simulink model "chap04"  (R2021a)
settings: Solver=FixedStepDiscrete  StartTime=0.0  StopTime=30  FixedStep=0.001  RelTol=1e-3
undefined symbols (not defined in the file): DiscIntNeverNeededParam
libraries: simulink x4
(part 6 of 7)

== system chap04/Subsystem/Subsystem7/Subsystem6 ==
  xx5 : Inport
  xx0 : Inport  Port=2
  xx3 : Inport  Port=3
  xx4 : Inport  Port=4
  vx5 : Inport  Port=5
  vx0 : Inport  Port=6
  vx3 : Inport  Port=7
  vx4 : Inport  Port=8
  Add : Sum
  Add1 : Sum  Inputs=-+
  Add10 : Sum  Inputs=-+
  Add2 : Sum  Inputs=+-
  Add4 : Sum  Inputs=-+
  Add5 : Sum  Inputs=+++
  Add6 : Sum  Inputs=+-
  Add8 : Sum  Inputs=+++
  Add9 : Sum  Inputs=+-
  Constant : Constant  Value=1.25
  Constant1 : Constant  Value=1.5
  Constant2 : Constant  Value=1.75
  Constant3 : Constant  Value=1.2
  Constant4 : Constant  Value=1.5
  Constant5 : Constant  Value=2.0
  Constant6 : Constant  Value=1.2
  Constant7 : Constant  Value=2.0
  Product{1,3..9} (8 alike) : Product
  utx : Outport
  wires:
  vx5/1 -> Add10/2, Add6/1, Add9/1
  vx4/1 -> Add10/1
  vx3/1 -> Add9/2
  xx3/1 -> Add2/2
  xx4/1 -> Add4/1
  Add/1 -> utx/1
  Add5/1 -> Product6/2
  Add2/1 -> Product5/1
  Product1/1 -> Add/2
  Constant2/1 -> Product1/1
  Constant/1 -> Product6/1
  Product6/1 -> Add/1
  Constant4/1 -> Product5/2
  xx5/1 -> Add1/2, Add4/2, Add2/1
  Add4/1 -> Product4/2
  Constant3/1 -> Product4/1
  Product5/1 -> Add5/3
  Product4/1 -> Add5/2
  Add8/1 -> Product1/2
  Constant6/1 -> Product8/1
  Add10/1 -> Product8/2
  Constant1/1 -> Product9/2
  Add9/1 -> Product9/1
  Product8/1 -> Add8/1
  Product9/1 -> Add8/2
  Constant7/1 -> Product3/1
  Add1/1 -> Product3/2
  xx0/1 -> Add1/1
  Product3/1 -> Add5/1
  Product7/1 -> Add8/3
  Add6/1 -> Product7/1
  Constant5/1 -> Product7/2
  vx0/1 -> Add6/2

== system chap04/Subsystem/Subsystem9/L+B ==
  Add : Sum
  Constant1 : Constant  Value=|
      | [2.7 0 0 0 0 0
      |      0 3.0 0 0 0 0
      |      0 0 3.0 0 0 0
      |      0 0 0 2.7 0 0
      |      0 0 0 0 2.7 0
      |      0 0 0 0 0 2.7]
  Constant2 : Constant  Value=|
      | [0.0 1.0 0.5 0.0 0.0 1.2
      |      1.0 0.0 0.0 0.5 0.0 1.5
      |      0.5 0.0 0.0 1.0 1.5 0.0
      |      0.0 0.5 1.0 0.0 1.2 0.0
      |      0.0 0.0 1.5 1.2 0.0 0.0
      |      1.2 1.5 0.0 0.0 0.0 0.0]
  Constant3 : Constant  Value=|
      | [0.0 0.0 0.0 0.0 0.0 0.0
      |      0.0 0.0 0.0 0.0 0.0 0.0
      |      0.0 0.0 0.0 0.0 0.0 0.0
      |      0.0 0.0 0.0 0.0 0.0 0.0
      |      0.0 0.0 0.0 0.0 2.0 0.0
      |      0.0 0.0 0.0 0.0 0.0 2.0]
  Subtract : Sum  Inputs=+-
  u : Outport
  wires:
  Constant2/1 -> Subtract/2
  Constant1/1 -> Subtract/1
  Subtract/1 -> Add/1
  Add/1 -> u/1
  Constant3/1 -> Add/2

== system chap04/Subsystem/Subsystem9/Subsystem1 ==
  xy3 : Inport
  xy1 : Inport  Port=2
  xy4 : Inport  Port=3
  xy5 : Inport  Port=4
  vy3 : Inport  Port=5
  vy1 : Inport  Port=6
  vy4 : Inport  Port=7
  vy5 : Inport  Port=8
  Add : Sum
  Add{1,4,6,8} (4 alike) : Sum  Inputs=-+
  Add2 : Sum  Inputs=+-
  Add5 : Sum  Inputs=+++
  Add7 : Sum  Inputs=+-
  Add9 : Sum  Inputs=+++
  Constant : Constant  Value=1.25
  Constant1 : Constant  Value=1.0
  Constant2 : Constant  Value=1.75
  Constant3 : Constant  Value=1.0
  Constant4 : Constant  Value=0.5
  Constant5 : Constant  Value=1.5
  Constant6 : Constant  Value=0.5
  Constant7 : Constant  Value=1.5
  Product{1,3..9} (8 alike) : Product
  p3y : Outport
  wires:
  Add9/1 -> Product1/2
  Product4/1 -> Add5/2
  Product5/1 -> Add5/3
  Constant3/1 -> Product4/1
  Add4/1 -> Product4/2
  xy3/1 -> Add1/2, Add4/2, Add2/1
  Constant4/1 -> Product5/2
  Product6/1 -> Add/1
  Constant/1 -> Product6/1
  Constant2/1 -> Product1/1
  Product1/1 -> Add/2
  Add2/1 -> Product5/1
  Add5/1 -> Product6/2
  Add/1 -> p3y/1
  xy4/1 -> Add4/1
  xy1/1 -> Add2/2
  xy5/1 -> Add1/1
  Constant5/1 -> Product3/1
  Add1/1 -> Product3/2
  Product3/1 -> Add5/1
  Product7/1 -> Add9/1
  Add6/1 -> Product7/2
  Constant7/1 -> Product7/1
  vy5/1 -> Add6/1
  vy1/1 -> Add7/2
  vy4/1 -> Add8/1
  Add7/1 -> Product9/1
  Constant6/1 -> Product9/2
  vy3/1 -> Add7/1, Add8/2, Add6/2
  Add8/1 -> Product8/2
  Constant1/1 -> Product8/1
  Product9/1 -> Add9/3
  Product8/1 -> Add9/2

== system chap04/Subsystem/Subsystem9/Subsystem2 ==
  xz3 : Inport
  xz1 : Inport  Port=2
  xz4 : Inport  Port=3
  xz5 : Inport  Port=4
  vz3 : Inport  Port=5
  vz1 : Inport  Port=6
  vz4 : Inport  Port=7
  vz5 : Inport  Port=8
  Add : Sum
  Add{1,4,6,8} (4 alike) : Sum  Inputs=-+
  Add2 : Sum  Inputs=+-
  Add5 : Sum  Inputs=+++
  Add7 : Sum  Inputs=+-
  Add9 : Sum  Inputs=+++
  Constant : Constant  Value=1.25
  Constant1 : Constant  Value=1.0
  Constant2 : Constant  Value=1.75
  Constant3 : Constant  Value=1.0
  Constant4 : Constant  Value=0.5
  Constant5 : Constant  Value=1.5
  Constant6 : Constant  Value=0.5
  Constant7 : Constant  Value=1.5
  Product{1,3..9} (8 alike) : Product
  p3z : Outport
  wires:
  Product8/1 -> Add9/2
  Product9/1 -> Add9/3
  Constant1/1 -> Product8/1
  Add8/1 -> Product8/2
  vz3/1 -> Add6/2, Add8/2, Add7/1
  Constant6/1 -> Product9/2
  Add7/1 -> Product9/1
  vz4/1 -> Add8/1
  vz1/1 -> Add7/2
  vz5/1 -> Add6/1
  Constant7/1 -> Product7/1
  Add6/1 -> Product7/2
  Product7/1 -> Add9/1
  Product3/1 -> Add5/1
  Add1/1 -> Product3/2
  Constant5/1 -> Product3/1
  xz5/1 -> Add1/1
  xz1/1 -> Add2/2
  xz4/1 -> Add4/1
  Add/1 -> p3z/1
  Add5/1 -> Product6/2
  Add2/1 -> Product5/1
  Product1/1 -> Add/2
  Constant2/1 -> Product1/1
  Constant/1 -> Product6/1
  Product6/1 -> Add/1
  Constant4/1 -> Product5/2
  xz3/1 -> Add2/1, Add4/2, Add1/2
  Add4/1 -> Product4/2
  Constant3/1 -> Product4/1
  Product5/1 -> Add5/3
  Product4/1 -> Add5/2
  Add9/1 -> Product1/2

== system chap04/Subsystem/Subsystem9/Subsystem3 ==
  xyk : Inport
  xy : Inport  Port=2
  vyk : Inport  Port=3
  vy : Inport  Port=4
  Add : Sum
  Add4 : Sum  Inputs=-+
  Add8 : Sum  Inputs=-+
  Constant : Constant  Value=1.25
  Constant1 : Constant  Value=1.75
  Product1 : Product
  Product6 : Product
  ey : Outport
  wires:
  vyk/1 -> Add8/2
  vy/1 -> Add8/1
  xy/1 -> Add4/1
  Add/1 -> ey/1
  Add4/1 -> Product6/2
  Product1/1 -> Add/2
  Constant1/1 -> Product1/1
  Constant/1 -> Product6/1
  Product6/1 -> Add/1
  xyk/1 -> Add4/2
  Add8/1 -> Product1/2

== system chap04/Subsystem/Subsystem9/Subsystem4 ==
  xzk : Inport
  xz : Inport  Port=2
  vzk : Inport  Port=3
  vz : Inport  Port=4
  Add : Sum
  Add4 : Sum  Inputs=-+
  Add8 : Sum  Inputs=-+
  Constant : Constant  Value=1.25
  Constant1 : Constant  Value=1.75
  Product1 : Product
  Product6 : Product
  ez : Outport
  wires:
  Add8/1 -> Product1/2
  xzk/1 -> Add4/2
  Product6/1 -> Add/1
  Constant/1 -> Product6/1
  Constant1/1 -> Product1/1
  Product1/1 -> Add/2
  Add4/1 -> Product6/2
  Add/1 -> ez/1
  xz/1 -> Add4/1
  vz/1 -> Add8/1
  vzk/1 -> Add8/2

== system chap04/Subsystem/Subsystem9/Subsystem5 ==
  xxk : Inport
  xx : Inport  Port=2
  vxk : Inport  Port=3
  vx : Inport  Port=4
  Add : Sum
  Add4 : Sum  Inputs=-+
  Add8 : Sum  Inputs=-+
  Constant : Constant  Value=1.25
  Constant1 : Constant  Value=1.75
  Product1 : Product
  Product6 : Product
  ex : Outport
  wires:
  Add8/1 -> Product1/2
  xxk/1 -> Add4/2
  Product6/1 -> Add/1
  Constant/1 -> Product6/1
  Constant1/1 -> Product1/1
  Product1/1 -> Add/2
  Add4/1 -> Product6/2
  Add/1 -> ex/1
  xx/1 -> Add4/1
  vx/1 -> Add8/1
  vxk/1 -> Add8/2

== system chap04/Subsystem/Subsystem9/Subsystem6 ==
  xx3 : Inport
  xx1 : Inport  Port=2
  xx4 : Inport  Port=3
  xx5 : Inport  Port=4
  vx3 : Inport  Port=5
  vx1 : Inport  Port=6
  vx4 : Inport  Port=7
  vx5 : Inport  Port=8
  Add : Sum
  Add{1,4,6,8} (4 alike) : Sum  Inputs=-+
  Add2 : Sum  Inputs=+-
  Add5 : Sum  Inputs=+++
  Add7 : Sum  Inputs=+-
  Add9 : Sum  Inputs=+++
  Constant : Constant  Value=1.25
  Constant1 : Constant  Value=1.0
  Constant2 : Constant  Value=1.75
  Constant3 : Constant  Value=1.0
  Constant4 : Constant  Value=0.5
  Constant5 : Constant  Value=1.5
  Constant6 : Constant  Value=0.5
  Constant7 : Constant  Value=1.5
  Product{1,3..9} (8 alike) : Product
  p3x : Outport
  wires:
  Product8/1 -> Add9/2
  Product9/1 -> Add9/3
  Constant1/1 -> Product8/1
  Add8/1 -> Product8/2
  vx3/1 -> Add6/2, Add8/2, Add7/1
  Constant6/1 -> Product9/2
  Add7/1 -> Product9/1
  vx4/1 -> Add8/1
  vx1/1 -> Add7/2
  vx5/1 -> Add6/1
  Constant7/1 -> Product7/1
  Add6/1 -> Product7/2
  Product7/1 -> Add9/1
  Product3/1 -> Add5/1
  Add1/1 -> Product3/2
  Constant5/1 -> Product3/1
  xx5/1 -> Add1/1
  xx1/1 -> Add2/2
  xx4/1 -> Add4/1
  Add/1 -> p3x/1
  Add5/1 -> Product6/2
  Add2/1 -> Product5/1
  Product1/1 -> Add/2
  Constant2/1 -> Product1/1
  Constant/1 -> Product6/1
  Product6/1 -> Add/1
  Constant4/1 -> Product5/2
  xx3/1 -> Add2/1, Add4/2, Add1/2
  Add4/1 -> Product4/2
  Constant3/1 -> Product4/1
  Product5/1 -> Add5/3
  Product4/1 -> Add5/2
  Add9/1 -> Product1/2

== system chap04/Subsystem1/Subsystem7/Subsystem1 ==
  Abs1 : Abs
  Add : Sum  Inputs=+++
  Constant : Constant  Value=0.8
  Constant1 : Constant  Value=0.1
  Constant3 : Constant  Value=0.1
  Delay1 : Delay
  Delay2 : Delay  DelayLength=1
  Product{1..4} (4 alike) : Product
  Random Number1 : RandomNumber  Mean=0.75  Variance=0.5  Seed=2  SampleTime=0.01
  Repeating Sequence Interpolated2 : simulink/Sources/Repeating Sequence Interpolated  OutValues=[0.5 0.25 0.4 0.35 0.1].'  TimeValues=[0 0.1 0.5 0.6 1].'  LookUpMeth=Use Input Nearest  tsamp=1  OutMin=[]  OutMax=[]  OutDataTypeStr=double  OutputDataTypeScalingMode=double  OutDataType=fixdt(0,8)  OutScaling=2^-10
  Scope : Scope
  Out2 : Outport
  wires:
  Delay1/1 -> Product2/1
  Delay2/1 -> Product1/1
  Constant/1 -> Product2/2
  Constant3/1 -> Product1/2
  Constant1/1 -> Product3/2
  Product3/1 -> Add/1
  Product1/1 -> Add/2
  Product2/1 -> Add/3
  Product4/1 -> Product3/1
  Add/1 -> Out2/1, Delay1/1, Delay2/1
  Abs1/1 -> Product4/1, Scope/1
  Random Number1/1 -> Abs1/1
  Repeating Sequence Interpolated2/1 -> Product4/2

== system chap04/Subsystem1/Subsystem7/Subsystem2 ==
  In2 : Inport
  Add : Sum  Inputs=+++
  Constant : Constant  Value=0.8
  Constant1 : Constant  Value=0.1
  Constant3 : Constant  Value=0.1
  Delay1 : Delay
  Delay2 : Delay  DelayLength=1
  Product1 : Product
  Product2 : Product
  Product3 : Product
  Out2 : Outport
  wires:
  Add/1 -> Delay2/1, Delay1/1, Out2/1
  In2/1 -> Product3/1
  Product2/1 -> Add/3
  Product1/1 -> Add/2
  Product3/1 -> Add/1
  Constant1/1 -> Product3/2
  Constant3/1 -> Product1/2
  Constant/1 -> Product2/2
  Delay2/1 -> Product1/1
  Delay1/1 -> Product2/1

== system chap04/Subsystem1/Subsystem7/Subsystem3 ==
  In2 : Inport
  Add : Sum  Inputs=+++
  Constant : Constant  Value=0.8
  Constant1 : Constant  Value=0.1
  Constant3 : Constant  Value=0.1
  Delay1 : Delay
  Delay2 : Delay  DelayLength=1
  Product1 : Product
  Product2 : Product
  Product3 : Product
  Out2 : Outport
  wires:
  Delay1/1 -> Product2/1
  Delay2/1 -> Product1/1
  Constant/1 -> Product2/2
  Constant3/1 -> Product1/2
  Constant1/1 -> Product3/2
  Product3/1 -> Add/1
  Product1/1 -> Add/2
  Product2/1 -> Add/3
  In2/1 -> Product3/1
  Add/1 -> Out2/1, Delay1/1, Delay2/1

== system chap04/Subsystem1/Subsystem7/Subsystem4 ==
  In2 : Inport
  Add : Sum  Inputs=+++
  Constant : Constant  Value=0.8
  Constant1 : Constant  Value=0.1
  Constant3 : Constant  Value=0.1
  Delay1 : Delay
  Delay2 : Delay  DelayLength=1
  Product1 : Product
  Product2 : Product
  Product3 : Product
  Out2 : Outport
  wires:
  Add/1 -> Delay2/1, Delay1/1, Out2/1
  In2/1 -> Product3/1
  Product2/1 -> Add/3
  Product1/1 -> Add/2
  Product3/1 -> Add/1
  Constant1/1 -> Product3/2
  Constant3/1 -> Product1/2
  Constant/1 -> Product2/2
  Delay2/1 -> Product1/1
  Delay1/1 -> Product2/1

== system chap04/Subsystem/Subsystem/Subsystem3/Subsystem ==
  e1 : Inport
  k3 : Inport  Port=2
  k4 : Inport  Port=3
  Add : Sum
  Constant3 : Constant  Value=-1
  Constant4 : Constant  Value=-1
  Discrete-Time Integrator1 : DiscreteIntegrator  SampleTime=-1  ICPrevOutput=DiscIntNeverNeededParam  ICPrevScaledInput=DiscIntNeverNeededParam
  Divide : Product  Inputs=*/
  MATLAB Function : MATLAB Function  TreatAsAtomicUnit=on
  Product3 : Product  Inputs=3
  Product5 : Product  Inputs=3
  z2 : Outport
  wires:
  Constant4/1 -> Product5/1
  Product5/1 -> Add/2
  Discrete-Time Integrator1/1 -> z2/1
  k3/1 -> Product3/3
  k4/1 -> Product5/3
  Divide/1 -> Add/1
  Add/1 -> Discrete-Time Integrator1/1
  Constant3/1 -> Product3/1
  e1/1 -> Product5/2, MATLAB Function/1(u), Product3/2
  MATLAB Function/1(y) -> Divide/2
  Product3/1 -> Divide/1

== system chap04/Subsystem/Subsystem/Subsystem3/Subsystem1 ==
  e1 : Inport
  k1 : Inport  Port=2
  Constant : Constant  Value=-1
  Divide : Product  Inputs=*/
  MATLAB Function : MATLAB Function  TreatAsAtomicUnit=on
  Product : Product  Inputs=3
  Out1 : Outport
  wires:
  e1/1 -> Product/2, MATLAB Function/1(u)
  Divide/1 -> Out1/1
  Constant/1 -> Product/1
  k1/1 -> Product/3
  MATLAB Function/1(y) -> Divide/2
  Product/1 -> Divide/1

== system chap04/Subsystem/Subsystem/Subsystem3/Subsystem2 ==
  e1 : Inport
  Constant1 : Constant  Value=0.2
  Discrete-Time Integrator1 : DiscreteIntegrator  gainval=1  InitialCondition=0.25  SampleTime=-1  ICPrevOutput=DiscIntNeverNeededParam  ICPrevScaledInput=DiscIntNeverNeededParam
  MATLAB Function : MATLAB Function  TreatAsAtomicUnit=on
  Product{,1..3,6} (5 alike) : Product
  Scope1 : Scope
  Sqrt : Sqrt  SaturateOnIntegerOverflow=on
  Square : Math  Operator=square  SaturateOnIntegerOverflow=on
  Subtract2 : Sum  Inputs=+-
  c1 : Constant  Value=0.3
  c2 : Constant  Value=0.3
  c3 : Constant  Value=0.5
  c4 : Constant  Value=0.5
  k1 : Outport
  k2 : Outport  Port=2
  k3 : Outport  Port=3
  k4 : Outport  Port=4
  wires:
  c2/1 -> Product/1
  Product/1 -> k2/1
  c3/1 -> Product1/1
  Product1/1 -> k3/1
  c4/1 -> Product2/1
  Product2/1 -> k4/1
  c1/1 -> Product3/1
  Product3/1 -> k1/1
  Sqrt/1 -> Product3/2
  Square/1 -> Product2/2
  e1/1 -> MATLAB Function/1(u)
  Product6/1 -> Subtract2/2
  MATLAB Function/1(y) -> Subtract2/1
  Subtract2/1 -> Discrete-Time Integrator1/1
  Constant1/1 -> Product6/1
  Discrete-Time Integrator1/1 -> Product6/2, Sqrt/1, Product/2, Square/1, Product1/2, Scope1/1

== system chap04/Subsystem/Subsystem/Subsystem3/Subsystem3 ==
  e1 : Inport
  k2 : Inport  Port=2
  Constant2 : Constant  Value=-1
  Product2 : Product  Inputs=3
  Out1 : Outport
  wires:
  Product2/1 -> Out1/1
  e1/1 -> Product2/2
  k2/1 -> Product2/3
  Constant2/1 -> Product2/1

== system chap04/Subsystem/Subsystem/Subsystem4/Subsystem ==
  zt3 : Inport
  Constant4 : Constant  Value=0
  Discrete-Time Integrator : DiscreteIntegrator  SampleTime=-1  UpperSaturationLimit=100  LowerSaturationLimit=-100  ICPrevOutput=DiscIntNeverNeededParam  ICPrevScaledInput=DiscIntNeverNeededParam
  Logical Operator : Logic  AllPortsSameDT=off  OutDataTypeStr=boolean
  MATLAB Function : MATLAB Function  TreatAsAtomicUnit=on
  Relational Operator : RelationalOperator  Operator===  OutDataTypeStr=boolean  RndMeth=Simplest
  Saturation : Saturate  UpperLimit=5  LowerLimit=-5
  Sign : Signum
  Sign1 : Signum
  Switch : Switch  Criteria=u2 > Threshold
  Out1 : Outport
  wires:
  MATLAB Function/1(y) -> Logical Operator/1
  Relational Operator/1 -> Logical Operator/2
  Constant4/1 -> Switch/1
  Sign1/1 -> Relational Operator/1
  zt3/1 -> Sign1/1, Switch/3
  Saturation/1 -> Out1/1, MATLAB Function/2(u2)
  Discrete-Time Integrator/1 -> Saturation/1, MATLAB Function/1(u1), Sign/1
  Sign/1 -> Relational Operator/2
  Logical Operator/1 -> Switch/2
  Switch/1 -> Discrete-Time Integrator/1

== system chap04/Subsystem/Subsystem/Subsystem7/Subsystem ==
  zt3 : Inport
  Constant4 : Constant  Value=0
  Discrete-Time Integrator : DiscreteIntegrator  SampleTime=-1  UpperSaturationLimit=100  LowerSaturationLimit=-100  ICPrevOutput=DiscIntNeverNeededParam  ICPrevScaledInput=DiscIntNeverNeededParam
  Logical Operator : Logic  AllPortsSameDT=off  OutDataTypeStr=boolean
  MATLAB Function : MATLAB Function  TreatAsAtomicUnit=on
  Relational Operator : RelationalOperator  Operator===  OutDataTypeStr=boolean  RndMeth=Simplest
  Saturation : Saturate  UpperLimit=5  LowerLimit=-5
  Sign : Signum
  Sign1 : Signum
  Switch : Switch  Criteria=u2 > Threshold
  Out1 : Outport
  wires:
  Switch/1 -> Discrete-Time Integrator/1
  Logical Operator/1 -> Switch/2
  Sign/1 -> Relational Operator/2
  Discrete-Time Integrator/1 -> Sign/1, MATLAB Function/1(u1), Saturation/1
  Saturation/1 -> MATLAB Function/2(u2), Out1/1
  zt3/1 -> Switch/3, Sign1/1
  Sign1/1 -> Relational Operator/1
  Constant4/1 -> Switch/1
  Relational Operator/1 -> Logical Operator/2
  MATLAB Function/1(y) -> Logical Operator/1

== system chap04/Subsystem/Subsystem/Subsystem8/Subsystem ==
  zt3 : Inport
  Constant4 : Constant  Value=0
  Discrete-Time Integrator : DiscreteIntegrator  SampleTime=-1  UpperSaturationLimit=100  LowerSaturationLimit=-100  ICPrevOutput=DiscIntNeverNeededParam  ICPrevScaledInput=DiscIntNeverNeededParam
  Logical Operator : Logic  AllPortsSameDT=off  OutDataTypeStr=boolean
  MATLAB Function : MATLAB Function  TreatAsAtomicUnit=on
  Relational Operator : RelationalOperator  Operator===  OutDataTypeStr=boolean  RndMeth=Simplest
  Saturation : Saturate  UpperLimit=5  LowerLimit=-5
  Sign : Signum
  Sign1 : Signum
  Switch : Switch  Criteria=u2 > Threshold
  Out1 : Outport
  wires:
  MATLAB Function/1(y) -> Logical Operator/1
  Relational Operator/1 -> Logical Operator/2
  Constant4/1 -> Switch/1
  Sign1/1 -> Relational Operator/1
  zt3/1 -> Sign1/1, Switch/3
  Saturation/1 -> Out1/1, MATLAB Function/2(u2)
  Discrete-Time Integrator/1 -> Saturation/1, MATLAB Function/1(u1), Sign/1
  Sign/1 -> Relational Operator/2
  Logical Operator/1 -> Switch/2
  Switch/1 -> Discrete-Time Integrator/1

== system chap04/Subsystem/Subsystem1/Subsystem3/Subsystem ==
  e1 : Inport
  k3 : Inport  Port=2
  k4 : Inport  Port=3
  Add : Sum
  Constant3 : Constant  Value=-1
  Constant4 : Constant  Value=-1
  Discrete-Time Integrator1 : DiscreteIntegrator  SampleTime=-1  ICPrevOutput=DiscIntNeverNeededParam  ICPrevScaledInput=DiscIntNeverNeededParam
  Divide : Product  Inputs=*/
  MATLAB Function : MATLAB Function  TreatAsAtomicUnit=on
  Product3 : Product  Inputs=3
  Product5 : Product  Inputs=3
  z2 : Outport
  wires:
  Constant4/1 -> Product5/1
  Product5/1 -> Add/2
  Discrete-Time Integrator1/1 -> z2/1
  k3/1 -> Product3/3
  k4/1 -> Product5/3
  Divide/1 -> Add/1
  Add/1 -> Discrete-Time Integrator1/1
  Constant3/1 -> Product3/1
  e1/1 -> Product5/2, MATLAB Function/1(u), Product3/2
  MATLAB Function/1(y) -> Divide/2
  Product3/1 -> Divide/1

== system chap04/Subsystem/Subsystem1/Subsystem3/Subsystem1 ==
  e1 : Inport
  k1 : Inport  Port=2
  Constant : Constant  Value=-1
  Divide : Product  Inputs=*/
  MATLAB Function : MATLAB Function  TreatAsAtomicUnit=on
  Product : Product  Inputs=3
  Out1 : Outport
  wires:
  e1/1 -> Product/2, MATLAB Function/1(u)
  Divide/1 -> Out1/1
  Constant/1 -> Product/1
  k1/1 -> Product/3
  MATLAB Function/1(y) -> Divide/2
  Product/1 -> Divide/1

== system chap04/Subsystem/Subsystem1/Subsystem3/Subsystem2 ==
  e1 : Inport
  Constant1 : Constant  Value=0.2
  Discrete-Time Integrator1 : DiscreteIntegrator  gainval=1  InitialCondition=0.25  SampleTime=-1  ICPrevOutput=DiscIntNeverNeededParam  ICPrevScaledInput=DiscIntNeverNeededParam
  MATLAB Function : MATLAB Function  TreatAsAtomicUnit=on
  Product{,1..3,6} (5 alike) : Product
  Scope1 : Scope
  Sqrt : Sqrt  SaturateOnIntegerOverflow=on
  Square : Math  Operator=square  SaturateOnIntegerOverflow=on
  Subtract2 : Sum  Inputs=+-
  c1 : Constant  Value=0.3
  c2 : Constant  Value=0.3
  c3 : Constant  Value=0.5
  c4 : Constant  Value=0.5
  k1 : Outport
  k2 : Outport  Port=2
  k3 : Outport  Port=3
  k4 : Outport  Port=4
  wires:
  c2/1 -> Product/1
  Product/1 -> k2/1
  c3/1 -> Product1/1
  Product1/1 -> k3/1
  c4/1 -> Product2/1
  Product2/1 -> k4/1
  c1/1 -> Product3/1
  Product3/1 -> k1/1
  Sqrt/1 -> Product3/2
  Square/1 -> Product2/2
  e1/1 -> MATLAB Function/1(u)
  Product6/1 -> Subtract2/2
  MATLAB Function/1(y) -> Subtract2/1
  Subtract2/1 -> Discrete-Time Integrator1/1
  Constant1/1 -> Product6/1
  Discrete-Time Integrator1/1 -> Product6/2, Sqrt/1, Product/2, Square/1, Product1/2, Scope1/1

== system chap04/Subsystem/Subsystem1/Subsystem3/Subsystem3 ==
  e1 : Inport
  k2 : Inport  Port=2
  Constant2 : Constant  Value=-1
  Product2 : Product  Inputs=3
  Out1 : Outport
  wires:
  Product2/1 -> Out1/1
  e1/1 -> Product2/2
  k2/1 -> Product2/3
  Constant2/1 -> Product2/1

== system chap04/Subsystem/Subsystem1/Subsystem4/Subsystem ==
  zt3 : Inport
  Constant4 : Constant  Value=0
  Discrete-Time Integrator : DiscreteIntegrator  SampleTime=-1  UpperSaturationLimit=100  LowerSaturationLimit=-100  ICPrevOutput=DiscIntNeverNeededParam  ICPrevScaledInput=DiscIntNeverNeededParam
  Logical Operator : Logic  AllPortsSameDT=off  OutDataTypeStr=boolean
  MATLAB Function : MATLAB Function  TreatAsAtomicUnit=on
  Relational Operator : RelationalOperator  Operator===  OutDataTypeStr=boolean  RndMeth=Simplest
  Saturation : Saturate  UpperLimit=5  LowerLimit=-5
  Sign : Signum
  Sign1 : Signum
  Switch : Switch  Criteria=u2 > Threshold
  Out1 : Outport
  wires:
  MATLAB Function/1(y) -> Logical Operator/1
  Relational Operator/1 -> Logical Operator/2
  Constant4/1 -> Switch/1
  Sign1/1 -> Relational Operator/1
  zt3/1 -> Sign1/1, Switch/3
  Saturation/1 -> Out1/1, MATLAB Function/2(u2)
  Discrete-Time Integrator/1 -> Saturation/1, MATLAB Function/1(u1), Sign/1
  Sign/1 -> Relational Operator/2
  Logical Operator/1 -> Switch/2
  Switch/1 -> Discrete-Time Integrator/1

== system chap04/Subsystem/Subsystem1/Subsystem7/Subsystem ==
  zt3 : Inport
  Constant4 : Constant  Value=0
  Discrete-Time Integrator : DiscreteIntegrator  SampleTime=-1  UpperSaturationLimit=100  LowerSaturationLimit=-100  ICPrevOutput=DiscIntNeverNeededParam  ICPrevScaledInput=DiscIntNeverNeededParam
  Logical Operator : Logic  AllPortsSameDT=off  OutDataTypeStr=boolean
  MATLAB Function : MATLAB Function  TreatAsAtomicUnit=on
  Relational Operator : RelationalOperator  Operator===  OutDataTypeStr=boolean  RndMeth=Simplest
  Saturation : Saturate  UpperLimit=5  LowerLimit=-5
  Sign : Signum
  Sign1 : Signum
  Switch : Switch  Criteria=u2 > Threshold
  Out1 : Outport
  wires:
  Switch/1 -> Discrete-Time Integrator/1
  Logical Operator/1 -> Switch/2
  Sign/1 -> Relational Operator/2
  Discrete-Time Integrator/1 -> Sign/1, MATLAB Function/1(u1), Saturation/1
  Saturation/1 -> MATLAB Function/2(u2), Out1/1
  zt3/1 -> Switch/3, Sign1/1
  Sign1/1 -> Relational Operator/1
  Constant4/1 -> Switch/1
  Relational Operator/1 -> Logical Operator/2
  MATLAB Function/1(y) -> Logical Operator/1

== system chap04/Subsystem/Subsystem1/Subsystem8/Subsystem ==
  zt3 : Inport
  Constant4 : Constant  Value=0
  Discrete-Time Integrator : DiscreteIntegrator  SampleTime=-1  UpperSaturationLimit=100  LowerSaturationLimit=-100  ICPrevOutput=DiscIntNeverNeededParam  ICPrevScaledInput=DiscIntNeverNeededParam
  Logical Operator : Logic  AllPortsSameDT=off  OutDataTypeStr=boolean
  MATLAB Function : MATLAB Function  TreatAsAtomicUnit=on
  Relational Operator : RelationalOperator  Operator===  OutDataTypeStr=boolean  RndMeth=Simplest
  Saturation : Saturate  UpperLimit=5  LowerLimit=-5
  Sign : Signum
  Sign1 : Signum
  Switch : Switch  Criteria=u2 > Threshold
  Out1 : Outport
  wires:
  MATLAB Function/1(y) -> Logical Operator/1
  Relational Operator/1 -> Logical Operator/2
  Constant4/1 -> Switch/1
  Sign1/1 -> Relational Operator/1
  zt3/1 -> Sign1/1, Switch/3
  Saturation/1 -> Out1/1, MATLAB Function/2(u2)
  Discrete-Time Integrator/1 -> Saturation/1, MATLAB Function/1(u1), Sign/1
  Sign/1 -> Relational Operator/2
  Logical Operator/1 -> Switch/2
  Switch/1 -> Discrete-Time Integrator/1

== system chap04/Subsystem/Subsystem2/Subsystem3/Subsystem ==
  e1 : Inport
  k3 : Inport  Port=2
  k4 : Inport  Port=3
  Add : Sum
  Constant3 : Constant  Value=-1
  Constant4 : Constant  Value=-1
  Discrete-Time Integrator1 : DiscreteIntegrator  SampleTime=-1  ICPrevOutput=DiscIntNeverNeededParam  ICPrevScaledInput=DiscIntNeverNeededParam
  Divide : Product  Inputs=*/
  MATLAB Function : MATLAB Function  TreatAsAtomicUnit=on
  Product3 : Product  Inputs=3
  Product5 : Product  Inputs=3
  z2 : Outport
  wires:
  Constant4/1 -> Product5/1
  Product5/1 -> Add/2
  Discrete-Time Integrator1/1 -> z2/1
  k3/1 -> Product3/3
  k4/1 -> Product5/3
  Divide/1 -> Add/1
  Add/1 -> Discrete-Time Integrator1/1
  Constant3/1 -> Product3/1
  e1/1 -> Product5/2, MATLAB Function/1(u), Product3/2
  MATLAB Function/1(y) -> Divide/2
  Product3/1 -> Divide/1

== system chap04/Subsystem/Subsystem2/Subsystem3/Subsystem1 ==
  e1 : Inport
  k1 : Inport  Port=2
  Constant : Constant  Value=-1
  Divide : Product  Inputs=*/
  MATLAB Function : MATLAB Function  TreatAsAtomicUnit=on
  Product : Product  Inputs=3
  Out1 : Outport
  wires:
  e1/1 -> Product/2, MATLAB Function/1(u)
  Divide/1 -> Out1/1
  Constant/1 -> Product/1
  k1/1 -> Product/3
  MATLAB Function/1(y) -> Divide/2
  Product/1 -> Divide/1

== system chap04/Subsystem/Subsystem2/Subsystem3/Subsystem2 ==
  e1 : Inport
  Constant1 : Constant  Value=0.2
  Discrete-Time Integrator1 : DiscreteIntegrator  gainval=1  InitialCondition=0.25  SampleTime=-1  ICPrevOutput=DiscIntNeverNeededParam  ICPrevScaledInput=DiscIntNeverNeededParam
  MATLAB Function : MATLAB Function  TreatAsAtomicUnit=on
  Product{,1..3,6} (5 alike) : Product
  Scope1 : Scope
  Sqrt : Sqrt  SaturateOnIntegerOverflow=on
  Square : Math  Operator=square  SaturateOnIntegerOverflow=on
  Subtract2 : Sum  Inputs=+-
  c1 : Constant  Value=0.3
  c2 : Constant  Value=0.3
  c3 : Constant  Value=0.5
  c4 : Constant  Value=0.5
  k1 : Outport
  k2 : Outport  Port=2
  k3 : Outport  Port=3
  k4 : Outport  Port=4
  wires:
  c2/1 -> Product/1
  Product/1 -> k2/1
  c3/1 -> Product1/1
  Product1/1 -> k3/1
  c4/1 -> Product2/1
  Product2/1 -> k4/1
  c1/1 -> Product3/1
  Product3/1 -> k1/1
  Sqrt/1 -> Product3/2
  Square/1 -> Product2/2
  e1/1 -> MATLAB Function/1(u)
  Product6/1 -> Subtract2/2
  MATLAB Function/1(y) -> Subtract2/1
  Subtract2/1 -> Discrete-Time Integrator1/1
  Constant1/1 -> Product6/1
  Discrete-Time Integrator1/1 -> Product6/2, Sqrt/1, Product/2, Square/1, Product1/2, Scope1/1

== system chap04/Subsystem/Subsystem2/Subsystem3/Subsystem3 ==
  e1 : Inport
  k2 : Inport  Port=2
  Constant2 : Constant  Value=-1
  Product2 : Product  Inputs=3
  Out1 : Outport
  wires:
  Product2/1 -> Out1/1
  e1/1 -> Product2/2
  k2/1 -> Product2/3
  Constant2/1 -> Product2/1

== system chap04/Subsystem/Subsystem2/Subsystem4/Subsystem ==
  zt3 : Inport
  Constant4 : Constant  Value=0
  Discrete-Time Integrator : DiscreteIntegrator  SampleTime=-1  UpperSaturationLimit=100  LowerSaturationLimit=-100  ICPrevOutput=DiscIntNeverNeededParam  ICPrevScaledInput=DiscIntNeverNeededParam
  Logical Operator : Logic  AllPortsSameDT=off  OutDataTypeStr=boolean
  MATLAB Function : MATLAB Function  TreatAsAtomicUnit=on
  Relational Operator : RelationalOperator  Operator===  OutDataTypeStr=boolean  RndMeth=Simplest
  Saturation : Saturate  UpperLimit=5  LowerLimit=-5
  Sign : Signum
  Sign1 : Signum
  Switch : Switch  Criteria=u2 > Threshold
  Out1 : Outport
  wires:
  MATLAB Function/1(y) -> Logical Operator/1
  Relational Operator/1 -> Logical Operator/2
  Constant4/1 -> Switch/1
  Sign1/1 -> Relational Operator/1
  zt3/1 -> Sign1/1, Switch/3
  Saturation/1 -> Out1/1, MATLAB Function/2(u2)
  Discrete-Time Integrator/1 -> Saturation/1, MATLAB Function/1(u1), Sign/1
  Sign/1 -> Relational Operator/2
  Logical Operator/1 -> Switch/2
  Switch/1 -> Discrete-Time Integrator/1

== system chap04/Subsystem/Subsystem2/Subsystem7/Subsystem ==
  zt3 : Inport
  Constant4 : Constant  Value=0
  Discrete-Time Integrator : DiscreteIntegrator  SampleTime=-1  UpperSaturationLimit=100  LowerSaturationLimit=-100  ICPrevOutput=DiscIntNeverNeededParam  ICPrevScaledInput=DiscIntNeverNeededParam
  Logical Operator : Logic  AllPortsSameDT=off  OutDataTypeStr=boolean
  MATLAB Function : MATLAB Function  TreatAsAtomicUnit=on
  Relational Operator : RelationalOperator  Operator===  OutDataTypeStr=boolean  RndMeth=Simplest
  Saturation : Saturate  UpperLimit=5  LowerLimit=-5
  Sign : Signum
  Sign1 : Signum
  Switch : Switch  Criteria=u2 > Threshold
  Out1 : Outport
  wires:
  Switch/1 -> Discrete-Time Integrator/1
  Logical Operator/1 -> Switch/2
  Sign/1 -> Relational Operator/2
  Discrete-Time Integrator/1 -> Sign/1, MATLAB Function/1(u1), Saturation/1
  Saturation/1 -> MATLAB Function/2(u2), Out1/1
  zt3/1 -> Switch/3, Sign1/1
  Sign1/1 -> Relational Operator/1
  Constant4/1 -> Switch/1
  Relational Operator/1 -> Logical Operator/2
  MATLAB Function/1(y) -> Logical Operator/1

== system chap04/Subsystem/Subsystem2/Subsystem8/Subsystem ==
  zt3 : Inport
  Constant4 : Constant  Value=0
  Discrete-Time Integrator : DiscreteIntegrator  SampleTime=-1  UpperSaturationLimit=100  LowerSaturationLimit=-100  ICPrevOutput=DiscIntNeverNeededParam  ICPrevScaledInput=DiscIntNeverNeededParam
  Logical Operator : Logic  AllPortsSameDT=off  OutDataTypeStr=boolean
  MATLAB Function : MATLAB Function  TreatAsAtomicUnit=on
  Relational Operator : RelationalOperator  Operator===  OutDataTypeStr=boolean  RndMeth=Simplest
  Saturation : Saturate  UpperLimit=5  LowerLimit=-5
  Sign : Signum
  Sign1 : Signum
  Switch : Switch  Criteria=u2 > Threshold
  Out1 : Outport
  wires:
  MATLAB Function/1(y) -> Logical Operator/1
  Relational Operator/1 -> Logical Operator/2
  Constant4/1 -> Switch/1
  Sign1/1 -> Relational Operator/1
  zt3/1 -> Sign1/1, Switch/3
  Saturation/1 -> Out1/1, MATLAB Function/2(u2)
  Discrete-Time Integrator/1 -> Saturation/1, MATLAB Function/1(u1), Sign/1
  Sign/1 -> Relational Operator/2
  Logical Operator/1 -> Switch/2
  Switch/1 -> Discrete-Time Integrator/1

== system chap04/Subsystem/Subsystem3/Subsystem3/Subsystem ==
  e1 : Inport
  k3 : Inport  Port=2
  k4 : Inport  Port=3
  Add : Sum
  Constant3 : Constant  Value=-1
  Constant4 : Constant  Value=-1
  Discrete-Time Integrator1 : DiscreteIntegrator  SampleTime=-1  ICPrevOutput=DiscIntNeverNeededParam  ICPrevScaledInput=DiscIntNeverNeededParam
  Divide : Product  Inputs=*/
  MATLAB Function : MATLAB Function  TreatAsAtomicUnit=on
  Product3 : Product  Inputs=3
  Product5 : Product  Inputs=3
  z2 : Outport
  wires:
  Constant4/1 -> Product5/1
  Product5/1 -> Add/2
  Discrete-Time Integrator1/1 -> z2/1
  k3/1 -> Product3/3
  k4/1 -> Product5/3
  Divide/1 -> Add/1
  Add/1 -> Discrete-Time Integrator1/1
  Constant3/1 -> Product3/1
  e1/1 -> Product5/2, MATLAB Function/1(u), Product3/2
  MATLAB Function/1(y) -> Divide/2
  Product3/1 -> Divide/1

== system chap04/Subsystem/Subsystem3/Subsystem3/Subsystem1 ==
  e1 : Inport
  k1 : Inport  Port=2
  Constant : Constant  Value=-1
  Divide : Product  Inputs=*/
  MATLAB Function : MATLAB Function  TreatAsAtomicUnit=on
  Product : Product  Inputs=3
  Out1 : Outport
  wires:
  e1/1 -> Product/2, MATLAB Function/1(u)
  Divide/1 -> Out1/1
  Constant/1 -> Product/1
  k1/1 -> Product/3
  MATLAB Function/1(y) -> Divide/2
  Product/1 -> Divide/1

== system chap04/Subsystem/Subsystem3/Subsystem3/Subsystem2 ==
  e1 : Inport
  Constant1 : Constant  Value=0.2
  Discrete-Time Integrator1 : DiscreteIntegrator  gainval=1  InitialCondition=0.25  SampleTime=-1  ICPrevOutput=DiscIntNeverNeededParam  ICPrevScaledInput=DiscIntNeverNeededParam
  MATLAB Function : MATLAB Function  TreatAsAtomicUnit=on
  Product{,1..3,6} (5 alike) : Product
  Scope1 : Scope
  Sqrt : Sqrt  SaturateOnIntegerOverflow=on
  Square : Math  Operator=square  SaturateOnIntegerOverflow=on
  Subtract2 : Sum  Inputs=+-
  c1 : Constant  Value=0.3
  c2 : Constant  Value=0.3
  c3 : Constant  Value=0.5
  c4 : Constant  Value=0.5
  k1 : Outport
  k2 : Outport  Port=2
  k3 : Outport  Port=3
  k4 : Outport  Port=4
  wires:
  c2/1 -> Product/1
  Product/1 -> k2/1
  c3/1 -> Product1/1
  Product1/1 -> k3/1
  c4/1 -> Product2/1
  Product2/1 -> k4/1
  c1/1 -> Product3/1
  Product3/1 -> k1/1
  Sqrt/1 -> Product3/2
  Square/1 -> Product2/2
  e1/1 -> MATLAB Function/1(u)
  Product6/1 -> Subtract2/2
  MATLAB Function/1(y) -> Subtract2/1
  Subtract2/1 -> Discrete-Time Integrator1/1
  Constant1/1 -> Product6/1
  Discrete-Time Integrator1/1 -> Product6/2, Sqrt/1, Product/2, Square/1, Product1/2, Scope1/1

== system chap04/Subsystem/Subsystem3/Subsystem3/Subsystem3 ==
  e1 : Inport
  k2 : Inport  Port=2
  Constant2 : Constant  Value=-1
  Product2 : Product  Inputs=3
  Out1 : Outport
  wires:
  Product2/1 -> Out1/1
  e1/1 -> Product2/2
  k2/1 -> Product2/3
  Constant2/1 -> Product2/1

== system chap04/Subsystem/Subsystem3/Subsystem4/Subsystem ==
  zt3 : Inport
  Constant4 : Constant  Value=0
  Discrete-Time Integrator : DiscreteIntegrator  SampleTime=-1  UpperSaturationLimit=100  LowerSaturationLimit=-100  ICPrevOutput=DiscIntNeverNeededParam  ICPrevScaledInput=DiscIntNeverNeededParam
  Logical Operator : Logic  AllPortsSameDT=off  OutDataTypeStr=boolean
  MATLAB Function : MATLAB Function  TreatAsAtomicUnit=on
  Relational Operator : RelationalOperator  Operator===  OutDataTypeStr=boolean  RndMeth=Simplest
  Saturation : Saturate  UpperLimit=5  LowerLimit=-5
  Sign : Signum
  Sign1 : Signum
  Switch : Switch  Criteria=u2 > Threshold
  Out1 : Outport
  wires:
  MATLAB Function/1(y) -> Logical Operator/1
  Relational Operator/1 -> Logical Operator/2
  Constant4/1 -> Switch/1
  Sign1/1 -> Relational Operator/1
  zt3/1 -> Sign1/1, Switch/3
  Saturation/1 -> Out1/1, MATLAB Function/2(u2)
  Discrete-Time Integrator/1 -> Saturation/1, MATLAB Function/1(u1), Sign/1
  Sign/1 -> Relational Operator/2
  Logical Operator/1 -> Switch/2
  Switch/1 -> Discrete-Time Integrator/1

== system chap04/Subsystem/Subsystem3/Subsystem7/Subsystem ==
  zt3 : Inport
  Constant4 : Constant  Value=0
  Discrete-Time Integrator : DiscreteIntegrator  SampleTime=-1  UpperSaturationLimit=100  LowerSaturationLimit=-100  ICPrevOutput=DiscIntNeverNeededParam  ICPrevScaledInput=DiscIntNeverNeededParam
  Logical Operator : Logic  AllPortsSameDT=off  OutDataTypeStr=boolean
  MATLAB Function : MATLAB Function  TreatAsAtomicUnit=on
  Relational Operator : RelationalOperator  Operator===  OutDataTypeStr=boolean  RndMeth=Simplest
  Saturation : Saturate  UpperLimit=5  LowerLimit=-5
  Sign : Signum
  Sign1 : Signum
  Switch : Switch  Criteria=u2 > Threshold
  Out1 : Outport
  wires:
  Switch/1 -> Discrete-Time Integrator/1
  Logical Operator/1 -> Switch/2
  Sign/1 -> Relational Operator/2
  Discrete-Time Integrator/1 -> Sign/1, MATLAB Function/1(u1), Saturation/1
  Saturation/1 -> MATLAB Function/2(u2), Out1/1
  zt3/1 -> Switch/3, Sign1/1
  Sign1/1 -> Relational Operator/1
  Constant4/1 -> Switch/1
  Relational Operator/1 -> Logical Operator/2
  MATLAB Function/1(y) -> Logical Operator/1

== system chap04/Subsystem/Subsystem3/Subsystem8/Subsystem ==
  zt3 : Inport
  Constant4 : Constant  Value=0
  Discrete-Time Integrator : DiscreteIntegrator  SampleTime=-1  UpperSaturationLimit=100  LowerSaturationLimit=-100  ICPrevOutput=DiscIntNeverNeededParam  ICPrevScaledInput=DiscIntNeverNeededParam
  Logical Operator : Logic  AllPortsSameDT=off  OutDataTypeStr=boolean
  MATLAB Function : MATLAB Function  TreatAsAtomicUnit=on
  Relational Operator : RelationalOperator  Operator===  OutDataTypeStr=boolean  RndMeth=Simplest
  Saturation : Saturate  UpperLimit=5  LowerLimit=-5
  Sign : Signum
  Sign1 : Signum
  Switch : Switch  Criteria=u2 > Threshold
  Out1 : Outport
  wires:
  MATLAB Function/1(y) -> Logical Operator/1
  Relational Operator/1 -> Logical Operator/2
  Constant4/1 -> Switch/1
  Sign1/1 -> Relational Operator/1
  zt3/1 -> Sign1/1, Switch/3
  Saturation/1 -> Out1/1, MATLAB Function/2(u2)
  Discrete-Time Integrator/1 -> Saturation/1, MATLAB Function/1(u1), Sign/1
  Sign/1 -> Relational Operator/2
  Logical Operator/1 -> Switch/2
  Switch/1 -> Discrete-Time Integrator/1

== system chap04/Subsystem/Subsystem4/Subsystem3/Subsystem ==
  e1 : Inport
  k3 : Inport  Port=2
  k4 : Inport  Port=3
  Add : Sum
  Constant3 : Constant  Value=-1
  Constant4 : Constant  Value=-1
  Discrete-Time Integrator1 : DiscreteIntegrator  SampleTime=-1  ICPrevOutput=DiscIntNeverNeededParam  ICPrevScaledInput=DiscIntNeverNeededParam
  Divide : Product  Inputs=*/
  MATLAB Function : MATLAB Function  TreatAsAtomicUnit=on
  Product3 : Product  Inputs=3
  Product5 : Product  Inputs=3
  z2 : Outport
  wires:
  Constant4/1 -> Product5/1
  Product5/1 -> Add/2
  Discrete-Time Integrator1/1 -> z2/1
  k3/1 -> Product3/3
  k4/1 -> Product5/3
  Divide/1 -> Add/1
  Add/1 -> Discrete-Time Integrator1/1
  Constant3/1 -> Product3/1
  e1/1 -> Product5/2, MATLAB Function/1(u), Product3/2
  MATLAB Function/1(y) -> Divide/2
  Product3/1 -> Divide/1

== system chap04/Subsystem/Subsystem4/Subsystem3/Subsystem1 ==
  e1 : Inport
  k1 : Inport  Port=2
  Constant : Constant  Value=-1
  Divide : Product  Inputs=*/
  MATLAB Function : MATLAB Function  TreatAsAtomicUnit=on
  Product : Product  Inputs=3
  Out1 : Outport
  wires:
  e1/1 -> Product/2, MATLAB Function/1(u)
  Divide/1 -> Out1/1
  Constant/1 -> Product/1
  k1/1 -> Product/3
  MATLAB Function/1(y) -> Divide/2
  Product/1 -> Divide/1

== system chap04/Subsystem/Subsystem4/Subsystem3/Subsystem2 ==
  e1 : Inport
  Constant1 : Constant  Value=0.2
  Discrete-Time Integrator1 : DiscreteIntegrator  gainval=1  InitialCondition=0.25  SampleTime=-1  ICPrevOutput=DiscIntNeverNeededParam  ICPrevScaledInput=DiscIntNeverNeededParam
  MATLAB Function : MATLAB Function  TreatAsAtomicUnit=on
  Product{,1..3,6} (5 alike) : Product
  Scope1 : Scope
  Sqrt : Sqrt  SaturateOnIntegerOverflow=on
  Square : Math  Operator=square  SaturateOnIntegerOverflow=on
  Subtract2 : Sum  Inputs=+-
  c1 : Constant  Value=0.3
  c2 : Constant  Value=0.3
  c3 : Constant  Value=0.5
  c4 : Constant  Value=0.5
  k1 : Outport
  k2 : Outport  Port=2
  k3 : Outport  Port=3
  k4 : Outport  Port=4
  wires:
  c2/1 -> Product/1
  Product/1 -> k2/1
  c3/1 -> Product1/1
  Product1/1 -> k3/1
  c4/1 -> Product2/1
  Product2/1 -> k4/1
  c1/1 -> Product3/1
  Product3/1 -> k1/1
  Sqrt/1 -> Product3/2
  Square/1 -> Product2/2
  e1/1 -> MATLAB Function/1(u)
  Product6/1 -> Subtract2/2
  MATLAB Function/1(y) -> Subtract2/1
  Subtract2/1 -> Discrete-Time Integrator1/1
  Constant1/1 -> Product6/1
  Discrete-Time Integrator1/1 -> Product6/2, Sqrt/1, Product/2, Square/1, Product1/2, Scope1/1

== system chap04/Subsystem/Subsystem4/Subsystem3/Subsystem3 ==
  e1 : Inport
  k2 : Inport  Port=2
  Constant2 : Constant  Value=-1
  Product2 : Product  Inputs=3
  Out1 : Outport
  wires:
  Product2/1 -> Out1/1
  e1/1 -> Product2/2
  k2/1 -> Product2/3
  Constant2/1 -> Product2/1

== system chap04/Subsystem/Subsystem4/Subsystem4/Subsystem ==
  zt3 : Inport
  Constant4 : Constant  Value=0
  Discrete-Time Integrator : DiscreteIntegrator  SampleTime=-1  UpperSaturationLimit=100  LowerSaturationLimit=-100  ICPrevOutput=DiscIntNeverNeededParam  ICPrevScaledInput=DiscIntNeverNeededParam
  Logical Operator : Logic  AllPortsSameDT=off  OutDataTypeStr=boolean
  MATLAB Function : MATLAB Function  TreatAsAtomicUnit=on
  Relational Operator : RelationalOperator  Operator===  OutDataTypeStr=boolean  RndMeth=Simplest
  Saturation : Saturate  UpperLimit=5  LowerLimit=-5
  Sign : Signum
  Sign1 : Signum
  Switch : Switch  Criteria=u2 > Threshold
  Out1 : Outport
  wires:
  MATLAB Function/1(y) -> Logical Operator/1
  Relational Operator/1 -> Logical Operator/2
  Constant4/1 -> Switch/1
  Sign1/1 -> Relational Operator/1
  zt3/1 -> Sign1/1, Switch/3
  Saturation/1 -> Out1/1, MATLAB Function/2(u2)
  Discrete-Time Integrator/1 -> Saturation/1, MATLAB Function/1(u1), Sign/1
  Sign/1 -> Relational Operator/2
  Logical Operator/1 -> Switch/2
  Switch/1 -> Discrete-Time Integrator/1

== system chap04/Subsystem/Subsystem4/Subsystem7/Subsystem ==
  zt3 : Inport
  Constant4 : Constant  Value=0
  Discrete-Time Integrator : DiscreteIntegrator  SampleTime=-1  UpperSaturationLimit=100  LowerSaturationLimit=-100  ICPrevOutput=DiscIntNeverNeededParam  ICPrevScaledInput=DiscIntNeverNeededParam
  Logical Operator : Logic  AllPortsSameDT=off  OutDataTypeStr=boolean
  MATLAB Function : MATLAB Function  TreatAsAtomicUnit=on
  Relational Operator : RelationalOperator  Operator===  OutDataTypeStr=boolean  RndMeth=Simplest
  Saturation : Saturate  UpperLimit=5  LowerLimit=-5
  Sign : Signum
  Sign1 : Signum
  Switch : Switch  Criteria=u2 > Threshold
  Out1 : Outport
  wires:
  Switch/1 -> Discrete-Time Integrator/1
  Logical Operator/1 -> Switch/2
  Sign/1 -> Relational Operator/2
  Discrete-Time Integrator/1 -> Sign/1, MATLAB Function/1(u1), Saturation/1
  Saturation/1 -> MATLAB Function/2(u2), Out1/1
  zt3/1 -> Switch/3, Sign1/1
  Sign1/1 -> Relational Operator/1
  Constant4/1 -> Switch/1
  Relational Operator/1 -> Logical Operator/2
  MATLAB Function/1(y) -> Logical Operator/1

== system chap04/Subsystem/Subsystem4/Subsystem8/Subsystem ==
  zt3 : Inport
  Constant4 : Constant  Value=0
  Discrete-Time Integrator : DiscreteIntegrator  SampleTime=-1  UpperSaturationLimit=100  LowerSaturationLimit=-100  ICPrevOutput=DiscIntNeverNeededParam  ICPrevScaledInput=DiscIntNeverNeededParam
  Logical Operator : Logic  AllPortsSameDT=off  OutDataTypeStr=boolean
  MATLAB Function : MATLAB Function  TreatAsAtomicUnit=on
  Relational Operator : RelationalOperator  Operator===  OutDataTypeStr=boolean  RndMeth=Simplest
  Saturation : Saturate  UpperLimit=5  LowerLimit=-5
  Sign : Signum
  Sign1 : Signum
  Switch : Switch  Criteria=u2 > Threshold
  Out1 : Outport
  wires:
  MATLAB Function/1(y) -> Logical Operator/1
  Relational Operator/1 -> Logical Operator/2
  Constant4/1 -> Switch/1
  Sign1/1 -> Relational Operator/1
  zt3/1 -> Sign1/1, Switch/3
  Saturation/1 -> Out1/1, MATLAB Function/2(u2)
  Discrete-Time Integrator/1 -> Saturation/1, MATLAB Function/1(u1), Sign/1
  Sign/1 -> Relational Operator/2
  Logical Operator/1 -> Switch/2
  Switch/1 -> Discrete-Time Integrator/1

== system chap04/Subsystem/Subsystem5/Subsystem3/Subsystem ==
  e1 : Inport
  k3 : Inport  Port=2
  k4 : Inport  Port=3
  Add : Sum
  Constant3 : Constant  Value=-1
  Constant4 : Constant  Value=-1
  Discrete-Time Integrator1 : DiscreteIntegrator  SampleTime=-1  ICPrevOutput=DiscIntNeverNeededParam  ICPrevScaledInput=DiscIntNeverNeededParam
  Divide : Product  Inputs=*/
  MATLAB Function : MATLAB Function  TreatAsAtomicUnit=on
  Product3 : Product  Inputs=3
  Product5 : Product  Inputs=3
  z2 : Outport
  wires:
  Constant4/1 -> Product5/1
  Product5/1 -> Add/2
  Discrete-Time Integrator1/1 -> z2/1
  k3/1 -> Product3/3
  k4/1 -> Product5/3
  Divide/1 -> Add/1
  Add/1 -> Discrete-Time Integrator1/1
  Constant3/1 -> Product3/1
  e1/1 -> Product5/2, MATLAB Function/1(u), Product3/2
  MATLAB Function/1(y) -> Divide/2
  Product3/1 -> Divide/1

== system chap04/Subsystem/Subsystem5/Subsystem3/Subsystem1 ==
  e1 : Inport
  k1 : Inport  Port=2
  Constant : Constant  Value=-1
  Divide : Product  Inputs=*/
  MATLAB Function : MATLAB Function  TreatAsAtomicUnit=on
  Product : Product  Inputs=3
  Out1 : Outport
  wires:
  e1/1 -> Product/2, MATLAB Function/1(u)
  Divide/1 -> Out1/1
  Constant/1 -> Product/1
  k1/1 -> Product/3
  MATLAB Function/1(y) -> Divide/2
  Product/1 -> Divide/1

== system chap04/Subsystem/Subsystem5/Subsystem3/Subsystem2 ==
  e1 : Inport
  Constant1 : Constant  Value=0.2
  Discrete-Time Integrator1 : DiscreteIntegrator  gainval=1  InitialCondition=0.25  SampleTime=-1  ICPrevOutput=DiscIntNeverNeededParam  ICPrevScaledInput=DiscIntNeverNeededParam
  MATLAB Function : MATLAB Function  TreatAsAtomicUnit=on
  Product{,1..3,6} (5 alike) : Product
  Scope1 : Scope
  Sqrt : Sqrt  SaturateOnIntegerOverflow=on
  Square : Math  Operator=square  SaturateOnIntegerOverflow=on
  Subtract2 : Sum  Inputs=+-
  c1 : Constant  Value=0.3
  c2 : Constant  Value=0.3
  c3 : Constant  Value=0.5
  c4 : Constant  Value=0.5
  k1 : Outport
  k2 : Outport  Port=2
  k3 : Outport  Port=3
  k4 : Outport  Port=4
  wires:
  c2/1 -> Product/1
  Product/1 -> k2/1
  c3/1 -> Product1/1
  Product1/1 -> k3/1
  c4/1 -> Product2/1
  Product2/1 -> k4/1
  c1/1 -> Product3/1
  Product3/1 -> k1/1
  Sqrt/1 -> Product3/2
  Square/1 -> Product2/2
  e1/1 -> MATLAB Function/1(u)
  Product6/1 -> Subtract2/2
  MATLAB Function/1(y) -> Subtract2/1
  Subtract2/1 -> Discrete-Time Integrator1/1
  Constant1/1 -> Product6/1
  Discrete-Time Integrator1/1 -> Product6/2, Sqrt/1, Product/2, Square/1, Product1/2, Scope1/1

== system chap04/Subsystem/Subsystem5/Subsystem3/Subsystem3 ==
  e1 : Inport
  k2 : Inport  Port=2
  Constant2 : Constant  Value=-1
  Product2 : Product  Inputs=3
  Out1 : Outport
  wires:
  Product2/1 -> Out1/1
  e1/1 -> Product2/2
  k2/1 -> Product2/3
  Constant2/1 -> Product2/1

== system chap04/Subsystem/Subsystem5/Subsystem4/Subsystem ==
  zt3 : Inport
  Constant4 : Constant  Value=0
  Discrete-Time Integrator : DiscreteIntegrator  SampleTime=-1  UpperSaturationLimit=100  LowerSaturationLimit=-100  ICPrevOutput=DiscIntNeverNeededParam  ICPrevScaledInput=DiscIntNeverNeededParam
  Logical Operator : Logic  AllPortsSameDT=off  OutDataTypeStr=boolean
  MATLAB Function : MATLAB Function  TreatAsAtomicUnit=on
  Relational Operator : RelationalOperator  Operator===  OutDataTypeStr=boolean  RndMeth=Simplest
  Saturation : Saturate  UpperLimit=5  LowerLimit=-5
  Sign : Signum
  Sign1 : Signum
  Switch : Switch  Criteria=u2 > Threshold
  Out1 : Outport
  wires:
  MATLAB Function/1(y) -> Logical Operator/1
  Relational Operator/1 -> Logical Operator/2
  Constant4/1 -> Switch/1
  Sign1/1 -> Relational Operator/1
  zt3/1 -> Sign1/1, Switch/3
  Saturation/1 -> Out1/1, MATLAB Function/2(u2)
  Discrete-Time Integrator/1 -> Saturation/1, MATLAB Function/1(u1), Sign/1
  Sign/1 -> Relational Operator/2
  Logical Operator/1 -> Switch/2
  Switch/1 -> Discrete-Time Integrator/1

== system chap04/Subsystem/Subsystem5/Subsystem7/Subsystem ==
  zt3 : Inport
  Constant4 : Constant  Value=0
  Discrete-Time Integrator : DiscreteIntegrator  SampleTime=-1  UpperSaturationLimit=100  LowerSaturationLimit=-100  ICPrevOutput=DiscIntNeverNeededParam  ICPrevScaledInput=DiscIntNeverNeededParam
  Logical Operator : Logic  AllPortsSameDT=off  OutDataTypeStr=boolean
  MATLAB Function : MATLAB Function  TreatAsAtomicUnit=on
  Relational Operator : RelationalOperator  Operator===  OutDataTypeStr=boolean  RndMeth=Simplest
  Saturation : Saturate  UpperLimit=5  LowerLimit=-5
  Sign : Signum
  Sign1 : Signum
  Switch : Switch  Criteria=u2 > Threshold
  Out1 : Outport
  wires:
  Switch/1 -> Discrete-Time Integrator/1
  Logical Operator/1 -> Switch/2
  Sign/1 -> Relational Operator/2
  Discrete-Time Integrator/1 -> Sign/1, MATLAB Function/1(u1), Saturation/1
  Saturation/1 -> MATLAB Function/2(u2), Out1/1
  zt3/1 -> Switch/3, Sign1/1
  Sign1/1 -> Relational Operator/1
  Constant4/1 -> Switch/1
  Relational Operator/1 -> Logical Operator/2
  MATLAB Function/1(y) -> Logical Operator/1

== system chap04/Subsystem/Subsystem5/Subsystem8/Subsystem ==
  zt3 : Inport
  Constant4 : Constant  Value=0
  Discrete-Time Integrator : DiscreteIntegrator  SampleTime=-1  UpperSaturationLimit=100  LowerSaturationLimit=-100  ICPrevOutput=DiscIntNeverNeededParam  ICPrevScaledInput=DiscIntNeverNeededParam
  Logical Operator : Logic  AllPortsSameDT=off  OutDataTypeStr=boolean
  MATLAB Function : MATLAB Function  TreatAsAtomicUnit=on
  Relational Operator : RelationalOperator  Operator===  OutDataTypeStr=boolean  RndMeth=Simplest
  Saturation : Saturate  UpperLimit=5  LowerLimit=-5
  Sign : Signum
  Sign1 : Signum
  Switch : Switch  Criteria=u2 > Threshold
  Out1 : Outport
  wires:
  MATLAB Function/1(y) -> Logical Operator/1
  Relational Operator/1 -> Logical Operator/2
  Constant4/1 -> Switch/1
  Sign1/1 -> Relational Operator/1
  zt3/1 -> Sign1/1, Switch/3
  Saturation/1 -> Out1/1, MATLAB Function/2(u2)
  Discrete-Time Integrator/1 -> Saturation/1, MATLAB Function/1(u1), Sign/1
  Sign/1 -> Relational Operator/2
  Logical Operator/1 -> Switch/2
  Switch/1 -> Discrete-Time Integrator/1

== matlab function chap04/Subsystem/Subsystem/Subsystem7/Subsystem/MATLAB Function ==
  data: u1 input; y output; u2 input
function y = fcn(u1,u2)


if (u1==u2)
    y = 0;
else
    y = 1;
end

== matlab function chap04/Subsystem/Subsystem/Subsystem8/Subsystem/MATLAB Function ==
  data: u1 input; y output; u2 input
function y = fcn(u1,u2)


if (u1==u2)
    y = 0;
else
    y = 1;
end

== matlab function chap04/Subsystem/Subsystem2/Subsystem12/MATLAB Function ==
  data: u input; y output
function y = fcn(u)

y = norm(u);

== matlab function chap04/Subsystem/Subsystem11/MATLAB Function ==
  data: u input; y output
function y = fcn(u)

y = norm(u);

== matlab function chap04/Subsystem/Subsystem11/MATLAB Function2 ==
  data: u input; y output
function y = fcn(u)

y = norm(u);

== matlab function chap04/Subsystem/Subsystem2/Subsystem4/Subsystem/MATLAB Function ==
  data: u1 input; y output; u2 input
function y = fcn(u1,u2)


if (u1==u2)
    y = 0;
else
    y = 1;
end

== matlab function chap04/Subsystem/Subsystem11/MATLAB Function3 ==
  data: u input; y output
function y = fcn(u)

y = norm(u);

== matlab function chap04/Subsystem/Subsystem7/MATLAB Function ==
  data: u input; y output
function y = fcn(u)

y = norm(u);

== matlab function chap04/Subsystem/Subsystem7/MATLAB Function2 ==
  data: u input; y output
function y = fcn(u)

y = norm(u);

== matlab function chap04/Subsystem/Subsystem7/MATLAB Function3 ==
  data: u input; y output
function y = fcn(u)

y = norm(u);
